simulink model "Labsession5"  (R2024b)
settings: Solver=VariableStepAuto  StartTime=0.0  StopTime=10.0  RelTol=1e-3
settings Model: Creator=Usuario_UMA  LastModifiedBy=Mountain
settings RTWCC: GPUComputeCapability=3.5

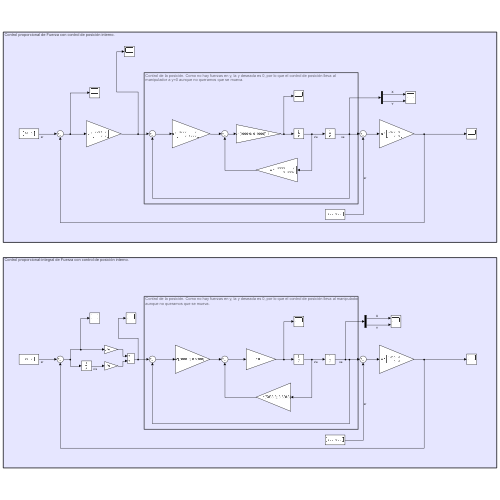
[thumbnail: Simulink's stored preview of the top-level diagram]
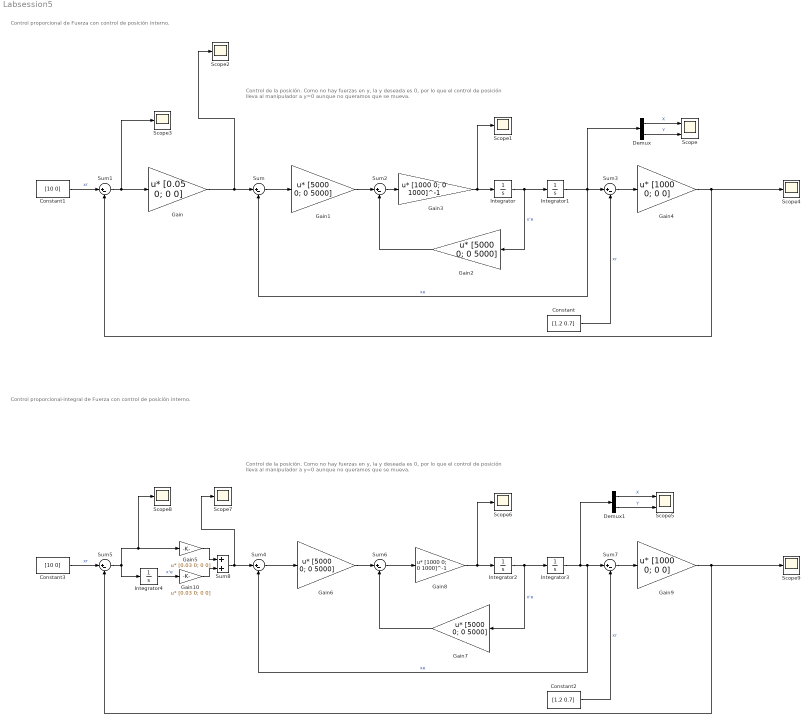
== system Labsession5 ==
  note: Control proporcional de Fuerza con control de posición interno.
  note: Control de la posición. Como no hay fuerzas en y, la y deseada es 0, por lo que el control de posición lleva al
      | manipulador a y=0 aunque no queramos que se mueva.
  note: Control proporcional-integral de Fuerza con control de posición interno.
  note: Control de la posición. Como no hay fuerzas en y, la y deseada es 0, por lo que el control de posición lleva al manipulador a y=0
      | aunque no queramos que se mueva.
  Constant : Constant  Value=[1.2 0.7]
  Constant1 : Constant  Value=[10 0]
  Constant2 : Constant  Value=[1.2 0.7]
  Constant3 : Constant  Value=[10 0]
  Demux : Demux  Outputs=2
  Demux1 : Demux  Outputs=2
  Gain : Gain  Gain=[0.05 0; 0 0]  Multiplication=Matrix(u*K)
  Gain{1..2,6..7} (4 alike) : Gain  Gain=[5000 0; 0 5000]  Multiplication=Matrix(u*K)
  Gain10 : Gain  Gain=[0.03 0; 0 0]  Multiplication=Matrix(u*K)
  Gain3 : Gain  Gain=[1000 0; 0 1000]^-1  Multiplication=Matrix(u*K)
  Gain4 : Gain  Gain=[1000 0; 0 0]  Multiplication=Matrix(u*K)
  Gain5 : Gain  Gain=[0.03 0; 0 0]  Multiplication=Matrix(u*K)
  Gain8 : Gain  Gain=[1000 0; 0 1000]^-1  Multiplication=Matrix(u*K)
  Gain9 : Gain  Gain=[1000 0; 0 0]  Multiplication=Matrix(u*K)
  Integrator : Integrator
  Integrator1 : Integrator  InitialCondition=[1.3 0.7]
  Integrator2 : Integrator
  Integrator3 : Integrator  InitialCondition=[1.3 0.7]
  Integrator4 : Integrator
  Scope : Scope  NumInputPorts=2
  Scope{1..4,6..9} (8 alike) : Scope
  Scope5 : Scope  NumInputPorts=2
  Sum{,1..7} (8 alike) : Sum  Inputs=|+-
  Sum8 : Sum
  wires:
  Gain/1 -> Scope2/1, Sum/1
  Sum/1 -> Gain1/1
  Sum1/1 -> Scope3/1, Gain/1
  Gain3/1 -> Integrator/1, Scope1/1
  Gain1/1 -> Sum2/1
  Sum2/1 -> Gain3/1
  Integrator/1 -> Gain2/1, Integrator1/1  "x'e"
  Gain2/1 -> Sum2/2
  Integrator1/1 -> Demux/1, Sum3/1, Sum/2  "xe"
  Constant/1 -> Sum3/2  "xr"
  Constant1/1 -> Sum1/1  "xr"
  Sum3/1 -> Gain4/1
  Gain4/1 -> Sum1/2, Scope4/1
  Gain9/1 -> Scope9/1, Sum5/2
  Sum7/1 -> Gain9/1
  Constant3/1 -> Sum5/1  "xr"
  Constant2/1 -> Sum7/2  "xr"
  Integrator3/1 -> Demux1/1, Sum4/2, Sum7/1  "xe"
  Gain7/1 -> Sum6/2
  Integrator2/1 -> Integrator3/1, Gain7/1  "x'e"
  Sum6/1 -> Gain8/1
  Gain6/1 -> Sum6/1
  Gain8/1 -> Integrator2/1, Scope6/1
  Sum5/1 -> Integrator4/1, Scope8/1, Gain5/1
  Sum4/1 -> Gain6/1
  Sum8/1 -> Scope7/1, Sum4/1
  Gain5/1 -> Sum8/1
  Integrator4/1 -> Gain10/1  "x'e"
  Gain10/1 -> Sum8/2
  Demux/1 -> Scope/1  "X"
  Demux/2 -> Scope/2  "Y"
  Demux1/1 -> Scope5/1  "X"
  Demux1/2 -> Scope5/2  "Y"
